simulink model "BKK5_y"  (Simulink 7.3)
settings: Solver=ode45  StartTime=0.0  StopTime=100  RelTol=1e-7
libraries: simulink x2
settings Model: Creator=Admin  LastModifiedBy=Sainquake
settings DebuggingCC: StrictBusMsg=ErrorLevel1

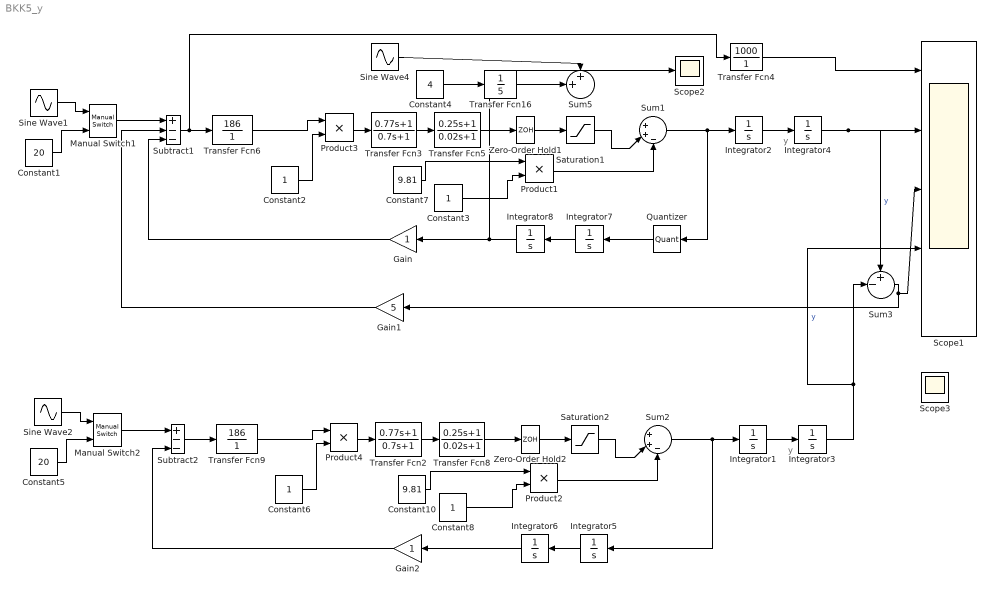
== system BKK5_y ==
  note: y
  note: y
  Constant1 : Constant  Value=20
  Constant10 : Constant  Value=9.81
  Constant{2..3,6,8} (4 alike) : Constant
  Constant4 : Constant  Value=4
  Constant5 : Constant  Value=20
  Constant7 : Constant  Value=9.81
  Gain : Gain  ParameterDataType=fixdt(1, 16)  ParameterScaling=2^0  OutDataType=fixdt(1, 16)  OutScaling=2^0
  Gain1 : Gain  Gain=5  ParameterDataType=fixdt(1, 16)  ParameterScaling=2^0  OutDataType=fixdt(1, 16)  OutScaling=2^0
  Gain2 : Gain  ParameterDataType=fixdt(1, 16)  ParameterScaling=2^0  OutDataType=fixdt(1, 16)  OutScaling=2^0
  Integrator{1..8} (8 alike) : Integrator
  Manual Switch1 : simulink/Signal Routing/Manual Switch  SystemSampleTime=-1  sw=0  action=0  varsize=off
  Manual Switch2 : simulink/Signal Routing/Manual Switch  SystemSampleTime=-1  sw=0  action=0  varsize=off
  Product{1..4} (4 alike) : Product  RndMeth=Zero
  Quantizer : Quantizer  QuantizationInterval=0.00390625  SampleTime=1/200
  Saturation1 : Saturate  UpperLimit=17.2  LowerLimit=-17.2
  Saturation2 : Saturate  UpperLimit=17.2  LowerLimit=-17.2
  Scope1 : Scope  NumInputPorts=5
      settings: YMin=-5~-5~-5~-5~-5  YMax=5~5~5~5~5  MaxDataPoints=500000
  Scope2 : Scope
      settings: YMin=4.916  YMax=4.927  SaveName=ScopeData2  MaxDataPoints=500000
  Scope3 : Scope  NumInputPorts=2
      settings: YMin=-5~-5  YMax=5~5  MaxDataPoints=500000
  Sine Wave1 : Sin  Amplitude=0.1  Bias=0  Frequency=0.628  Phase=0  Samples=10  SampleTime=0  Offset=0
  Sine Wave2 : Sin  Amplitude=0.1  Bias=0  Frequency=0.628  Phase=0  Samples=10  SampleTime=0  Offset=0
  Sine Wave4 : Sin  Amplitude=0.3  Bias=0  Frequency=0.3  Phase=1.57  Samples=10  SampleTime=0  Offset=0
  Subtract1 : Sum  Inputs=+--
  Subtract2 : Sum  Inputs=+--
  Sum1 : Sum  Inputs=|++-
  Sum2 : Sum  Inputs=|++-
  Sum3 : Sum  Inputs=+-|
  Sum5 : Sum  Inputs=++|
  Transfer Fcn16 : TransferFcn  Denominator=[ 5 ]
  Transfer Fcn2 : TransferFcn  Numerator=[0.77 1]  Denominator="[0.7  1]"
  Transfer Fcn3 : TransferFcn  Numerator=[0.77 1]  Denominator="[0.7  1]"
  Transfer Fcn4 : TransferFcn  Numerator=[1000]  Denominator=[ 1 ]
  Transfer Fcn5 : TransferFcn  Numerator=[0.25 1]  Denominator="[0.02  1]"
  Transfer Fcn6 : TransferFcn  Numerator=186  Denominator=[ 1 ]
  Transfer Fcn8 : TransferFcn  Numerator=[0.25 1]  Denominator="[0.02  1]"
  Transfer Fcn9 : TransferFcn  Numerator=186  Denominator=[ 1 ]
  Zero-Order Hold1 : ZeroOrderHold  SampleTime=1/200
  Zero-Order Hold2 : ZeroOrderHold  SampleTime=1/200
  wires:
  Subtract1/1 -> Transfer Fcn6/1, Transfer Fcn4/1
  Transfer Fcn3/1 -> Transfer Fcn5/1
  Integrator2/1 -> Integrator4/1
  Constant1/1 -> Manual Switch1/2
  Integrator4/1 -> Scope1/2, Sum3/1  "y"
  Sum1/1 -> Integrator2/1, Quantizer/1
  Transfer Fcn5/1 -> Zero-Order Hold1/1
  Constant4/1 -> Transfer Fcn16/1
  Sine Wave1/1 -> Manual Switch1/1
  Constant3/1 -> Product1/2
  Constant7/1 -> Product1/1
  Constant2/1 -> Product3/2
  Product3/1 -> Transfer Fcn3/1
  Transfer Fcn6/1 -> Product3/1
  Zero-Order Hold1/1 -> Saturation1/1
  Saturation1/1 -> Sum1/2
  Transfer Fcn16/1 -> Sum5/2
  Sine Wave4/1 -> Sum5/1
  Gain/1 -> Subtract1/3
  Integrator7/1 -> Integrator8/1
  Manual Switch1/1 -> Subtract1/1
  Integrator8/1 -> Gain/1, Scope2/1
  Transfer Fcn4/1 -> Scope1/1
  Product1/1 -> Sum1/3
  Quantizer/1 -> Integrator7/1
  Subtract2/1 -> Transfer Fcn9/1
  Transfer Fcn2/1 -> Transfer Fcn8/1
  Integrator1/1 -> Integrator3/1
  Constant5/1 -> Manual Switch2/2
  Integrator3/1 -> Sum3/2, Scope1/4  "y"
  Sum2/1 -> Integrator1/1, Integrator5/1
  Transfer Fcn8/1 -> Zero-Order Hold2/1
  Sine Wave2/1 -> Manual Switch2/1
  Constant8/1 -> Product2/2
  Constant10/1 -> Product2/1
  Constant6/1 -> Product4/2
  Product4/1 -> Transfer Fcn2/1
  Transfer Fcn9/1 -> Product4/1
  Zero-Order Hold2/1 -> Saturation2/1
  Saturation2/1 -> Sum2/2
  Gain2/1 -> Subtract2/3
  Integrator5/1 -> Integrator6/1
  Manual Switch2/1 -> Subtract2/1
  Integrator6/1 -> Gain2/1
  Product2/1 -> Sum2/3
  Sum3/1 -> Gain1/1, Scope1/3
  Gain1/1 -> Subtract1/2
